simulink model "fft_wideband_real"  (R2012b)
settings: Solver=ode45  StartTime=0.0  StopTime=19999  RelTol=1e-3
undefined symbols (not defined in the file): fft_wideband_real_shift_schedule_user_data_out
libraries: xbsIndex_r4 x8703, xbsReplacements_r4 x36, xps_library x24, dspsigops x16, simulink_xsg_bridge x1
(part 9 of 51)

== system fft_wideband_real/fft_wideband_real/phase_mult/phase3_coeffs ==
  rst : Inport
  Counter : xbsIndex_r4/Counter  cnt_type=Free Running  cnt_to=Inf  operation=Up  start_count=0  cnt_by_val=1  arith_type=Unsigned  n_bits=6  bin_pt=0  load_pin=off  rst=on  en=off  explicit_period=on  period=1  dbl_ovrd=off  use_behavioral_HDL=off  implementation=Fabric  block_type=counter
  Slice : xbsIndex_r4/Slice  nbits=6  boolean_output=off  mode=Upper Bit Location + Width  bit1=0  base1=MSB of Input  bit0=0  base0=LSB of Input  dbl_ovrd=off  block_type=slice
  bram_din_const : xbsIndex_r4/Constant  const=0  gui_display_data_type=Fixed-point  arith_type=Signed (2's comp)  n_bits=18  bin_pt=17  preci_type=Single  exp_width=8  frac_width=24  explicit_period=off  period=1  equ=P=C  opselect=C  inp2=PCIN>>17  opr=+  inp1=P  carry=CIN  dbl_ovrd=off  block_type=constant
  bram_we_const : xbsIndex_r4/Constant  const=0  gui_display_data_type=Fixed-point  arith_type=Boolean  n_bits=16  bin_pt=14  preci_type=Single  exp_width=8  frac_width=24  explicit_period=off  period=1  equ=P=C  opselect=C  inp2=PCIN>>17  opr=+  inp1=P  carry=CIN  dbl_ovrd=off  block_type=constant
  cnt_sign_exta : xbsIndex_r4/Convert  gui_display_data_type=Fixed-point  arith_type=Unsigned  n_bits=10  bin_pt=0  float_type=Single  exp_bits=8  fraction_bits=24  quantization=Truncate  overflow=Wrap  en=off  latency=0  dbl_ovrd=off  pipeline=off  block_type=convert
  cnt_sign_extb : xbsIndex_r4/Convert  gui_display_data_type=Fixed-point  arith_type=Unsigned  n_bits=9  bin_pt=0  float_type=Single  exp_bits=8  fraction_bits=24  quantization=Truncate  overflow=Wrap  en=off  latency=0  dbl_ovrd=off  pipeline=off  block_type=convert
  coeff_mem : xbsIndex_r4/Dual Port RAM  depth=1024  initVector=[1 0.999923706054688 0.999702453613281 0.999320983886719 0.998794555664062 0.998115539550781 0.997291564941406 0.996315002441406 0.995185852050781 0.993904113769531 0.992477416992188 0.99090576171875 0.989173889160156 0.9873046875 0.985275268554688 0.983108520507812 0.980781555175781 0.978317260742188 0.975700378417969 0.972938537597656 0.97003173828125 0.96697998046875 0.963775634765625 0.960433959960938 0.956939697265625 0.95330810546875 0.949531555175781 0.945610046386719 0.941543579101562 0.937339782714844 0.932991027832031 0.928504943847656 0.923881530761719 0.919113159179688 0.914207458496094 0.909164428710938 0.90399169921875 0.898674011230469 0.893226623535156 0.887641906738281 0.881919860839844 0.876068115234375 0.870086669921875 0.863975524902344 0.85772705078125 0.851356506347656 0.844856262207031 0.838226318359375 0.831466674804688 0.824592590332031 0.817581176757812 0.810455322265625 0.803207397460938 0.79583740234375 0.788345336914062 0.780738830566406 0.77301025390625 0.765167236328125 0.757209777832031 0.749137878417969 0.740951538085938 0.732650756835938 0.724250793457031 0.715728759765625 0 0 0 0 0 0 0 0 0 0 0 0 0 0 0 0 0 0 0 0 0 0 0 0 0 0 0 0 0 0 0 0 0 0 0 0 0 0 0 0 0 0 0 0 0 0 0 0 0 0 0 0 0 0 0 0 0 0 0 0 0 0 0 0 0 0 0 0 0 0 0 0 0 0 0 0 0 0 0 0 0 0 0 0 0 0 0 0 0 0 0 0 0 0 0 0 0 0 0 0 0 0 0 0 0 0 0 0 0 0 0 0 0 0 0 0 0 0 0 0 0 0 0 0 0 0 0 0 0 0 0 0 0 0 0 0 0 0 0 0 0 0 0 0 0 0 0 0 0 0 0 0 0 0 0 0 0 0 0 0 0 0 0 0 0 0 0 0 0 0 0 0 0 0 0 0 0 0 0 0 0 0 0 0 0 0 0 0 0 0 0 0 0 0 0 0 0 0 0 0 0 0 0 0 0 0 0 0 0 0 0 0 0 0 0 0 0 0 0 0 0 0 0 0 0 0 0 0 0 0 0 0 0 0 0 0 0 0 0 0 0 0 0 0 0 0 0 0 0 0 0 0 0 0 0 0 0 0 0 0 0 0 0 0 0 0 0 0 0 0 0 0 0 0 0 0 0 0 0 0 0 0 0 0 0 0 0 0 0 0 0 0 0 0 0 0 0 0 0 0 0 0 0 0 0 0 0 0 0 0 0 0 0 0 0 0 0 0 0 0 0 0 0 0 0 0 0 0 0 0 0 0 0 0 0 0 0 0 0 0 0 0 0 0 0 0 0 0 0 0 0 0 0 0 0 0 0 0 0 0 0 0 0 0 0 0 0 0 0 0 0 0 0 0 0 0 0 0 0 0 0 0 0 0 0 0 0 0 0 0 0 0 0 0 0 0 0 0 0 0 0 0 0 0 0 0 0 0 0 0 0 0 0 0 0 0 0 0 0 0 0 0 0 0 0 0 0 0 0 0 0 0 0 0 0 0 0 0 0 0 0 0 0 0 0 0 0 0 0 -0.01226806640625 -0.0245437622070312 -0.03680419921875 -0.0490646362304688 -0.0613174438476562 -0.0735626220703125 -0.0858001708984375 -0.0980148315429688 -0.110221862792969 -0.122413635253906 -0.13458251953125 -0.146728515625 -0.158859252929688 -0.17095947265625 -0.183036804199219 -0.195091247558594 -0.207115173339844 -0.219100952148438 -0.231056213378906 -0.24298095703125 -0.254867553710938 -0.266716003417969 -0.278518676757812 -0.290283203125 -0.302009582519531 -0.313682556152344 -0.325309753417969 -0.336891174316406 -0.348419189453125 -0.359893798828125 -0.371315002441406 -0.382682800292969 -0.393989562988281 -0.405242919921875 -0.416427612304688 -0.427558898925781 -0.438613891601562 -0.449607849121094 -0.460540771484375 -0.471397399902344 -0.482185363769531 -0.492897033691406 -0.5035400390625 -0.51409912109375 -0.524589538574219 -0.534996032714844 -0.545326232910156 -0.555572509765625 -0.56573486328125 -0.5758056640625 -0.585800170898438 -0.595695495605469 -0.605514526367188 -0.615234375 -0.624862670898438 -0.634391784667969 -0.643829345703125 -0.653175354003906 -0.66241455078125 -0.671562194824219 -0.68060302734375 -0.689537048339844 -0.698379516601562 0 0 0 0 0 0 0 0 0 0 0 0 0 0 0 0 0 0 0 0 0 0 0 0 0 0 0 0 0 0 0 0 0 0 0 0 0 0 0 0 0 0 0 0 0 0 0 0 0 0 0 0 0 0 0 0 0 0 0 0 0 0 0 0 0 0 0 0 0 0 0 0 0 0 0 0 0 0 0 0 0 0 0 0 0 0 0 0 0 0 0 0 0 0 0 0 0 0 0 0 0 0 0 0 0 0 0 0 0 0 0 0 0 0 0 0 0 0 0 0 0 0 0 0 0 0 0 0 0 0 0 0 0 0 0 0 0 0 0 0 0 0 0 0 0 0 0 0 0 0 0 0 0 0 0 0 0 0 0 0 0 0 0 0 0 0 0 0 0 0 0 0 0 0 0 0 0 0 0 0 0 0 0 0 0 0 0 0 0 0 0 0 0 0 0 0 0 0 0 0 0 0 0 0 0 0 0 0 0 0 0 0 0 0 0 0 0 0 0 0 0 0 0 0 0 0 0 0 0 0 0 0 0 0 0 0 0 0 0 0 0 0 0 0 0 0 0 0 0 0 0 0 0 0 0 0 0 0 0 0 0 0 0 0 0 0 0 0 0 0 0 0 0 0 0 0 0 0 0 0 0 0 0 0 0 0 0 0 0 0 0 0 0 0 0 0 0 0 0 0 0 0 0 0 0 0 0 0 0 0 0 0 0 0 0 0 0 0 0 0 0 0 0 0 0 0 0 0 0 0 0 0 0 0 0 0 0 0 0 0 0 0 0 0 0 0 0 0 0 0 0 0 0 0 0 0 0 0 0 0 0 0 0 0 0 0 0 0 0 0 0 0 0 0 0 0 0 0 0 0 0 0 0 0 0 0 0 0 0 0 0 0 0 0 0 0 0 0 0 0 0 0 0 0 0 0 0 0 0 0 0 0 0 0 0 0 0 0 0 0 0 0 0 0 0 0 0 0 0 0 0 0 0 0 0 0 0 0 0 0 0 0 0 0 0 0 0 0]  distributed_mem=Block RAM  init_a=0  init_b=0  rst_a=off  rst_b=off  en_a=off  en_b=off  latency=2  write_mode_A=Read After Write  write_mode_B=Read After Write  dbl_ovrd=off  optimize=Area  use_rpm=on  block_type=dpram
  counter_b_concat : xbsIndex_r4/Concat  num_inputs=2  dbl_ovrd=off  block_type=concat
  counter_b_pad : xbsIndex_r4/Constant  const=1  gui_display_data_type=Fixed-point  arith_type=Unsigned  n_bits=1  bin_pt=0  preci_type=Single  exp_width=8  frac_width=24  explicit_period=off  period=1  equ=P=C  opselect=C  inp2=PCIN>>17  opr=+  inp1=P  carry=CIN  dbl_ovrd=off  block_type=constant
  ri_to_c : Subsystem
  w : Outport
  wires:
  Slice/1 -> cnt_sign_extb/1, cnt_sign_exta/1
  bram_din_const/1 -> coeff_mem/5, coeff_mem/2
  bram_we_const/1 -> coeff_mem/6, coeff_mem/3
  ri_to_c/1(c) -> w/1
  coeff_mem/2 -> ri_to_c/2(im)
  coeff_mem/1 -> ri_to_c/1(re)
  counter_b_concat/1 -> coeff_mem/4
  cnt_sign_exta/1 -> coeff_mem/1
  cnt_sign_extb/1 -> counter_b_concat/2
  counter_b_pad/1 -> counter_b_concat/1
  Counter/1 -> Slice/1
  rst/1 -> Counter/1

== system fft_wideband_real/fft_wideband_real/phase_mult/phase4_coeffs ==
  rst : Inport
  Counter : xbsIndex_r4/Counter  cnt_type=Free Running  cnt_to=Inf  operation=Up  start_count=0  cnt_by_val=1  arith_type=Unsigned  n_bits=6  bin_pt=0  load_pin=off  rst=on  en=off  explicit_period=on  period=1  dbl_ovrd=off  use_behavioral_HDL=off  implementation=Fabric  block_type=counter
  Slice : xbsIndex_r4/Slice  nbits=6  boolean_output=off  mode=Upper Bit Location + Width  bit1=0  base1=MSB of Input  bit0=0  base0=LSB of Input  dbl_ovrd=off  block_type=slice
  bram_din_const : xbsIndex_r4/Constant  const=0  gui_display_data_type=Fixed-point  arith_type=Signed (2's comp)  n_bits=18  bin_pt=17  preci_type=Single  exp_width=8  frac_width=24  explicit_period=off  period=1  equ=P=C  opselect=C  inp2=PCIN>>17  opr=+  inp1=P  carry=CIN  dbl_ovrd=off  block_type=constant
  bram_we_const : xbsIndex_r4/Constant  const=0  gui_display_data_type=Fixed-point  arith_type=Boolean  n_bits=16  bin_pt=14  preci_type=Single  exp_width=8  frac_width=24  explicit_period=off  period=1  equ=P=C  opselect=C  inp2=PCIN>>17  opr=+  inp1=P  carry=CIN  dbl_ovrd=off  block_type=constant
  cnt_sign_exta : xbsIndex_r4/Convert  gui_display_data_type=Fixed-point  arith_type=Unsigned  n_bits=10  bin_pt=0  float_type=Single  exp_bits=8  fraction_bits=24  quantization=Truncate  overflow=Wrap  en=off  latency=0  dbl_ovrd=off  pipeline=off  block_type=convert
  cnt_sign_extb : xbsIndex_r4/Convert  gui_display_data_type=Fixed-point  arith_type=Unsigned  n_bits=9  bin_pt=0  float_type=Single  exp_bits=8  fraction_bits=24  quantization=Truncate  overflow=Wrap  en=off  latency=0  dbl_ovrd=off  pipeline=off  block_type=convert
  coeff_mem : xbsIndex_r4/Dual Port RAM  depth=1024  initVector=[1 0.999832153320312 0.999320983886719 0.99847412109375 0.997291564941406 0.995765686035156 0.993904113769531 0.991706848144531 0.989173889160156 0.986305236816406 0.983108520507812 0.979568481445312 0.975700378417969 0.971504211425781 0.96697998046875 0.962120056152344 0.956939697265625 0.951431274414062 0.945610046386719 0.939460754394531 0.932991027832031 0.92620849609375 0.919113159179688 0.911705017089844 0.90399169921875 0.895965576171875 0.887641906738281 0.879013061523438 0.870086669921875 0.860870361328125 0.851356506347656 0.841552734375 0.831466674804688 0.82110595703125 0.810455322265625 0.799537658691406 0.788345336914062 0.776885986328125 0.765167236328125 0.753189086914062 0.740951538085938 0.728462219238281 0.715728759765625 0.702751159667969 0.689537048339844 0.676094055175781 0.66241455078125 0.648513793945312 0.634391784667969 0.62005615234375 0.605514526367188 0.59075927734375 0.5758056640625 0.560661315917969 0.545326232910156 0.529800415039062 0.51409912109375 0.49822998046875 0.482185363769531 0.465972900390625 0.449607849121094 0.433090209960938 0.416427612304688 0.399627685546875 0 0 0 0 0 0 0 0 0 0 0 0 0 0 0 0 0 0 0 0 0 0 0 0 0 0 0 0 0 0 0 0 0 0 0 0 0 0 0 0 0 0 0 0 0 0 0 0 0 0 0 0 0 0 0 0 0 0 0 0 0 0 0 0 0 0 0 0 0 0 0 0 0 0 0 0 0 0 0 0 0 0 0 0 0 0 0 0 0 0 0 0 0 0 0 0 0 0 0 0 0 0 0 0 0 0 0 0 0 0 0 0 0 0 0 0 0 0 0 0 0 0 0 0 0 0 0 0 0 0 0 0 0 0 0 0 0 0 0 0 0 0 0 0 0 0 0 0 0 0 0 0 0 0 0 0 0 0 0 0 0 0 0 0 0 0 0 0 0 0 0 0 0 0 0 0 0 0 0 0 0 0 0 0 0 0 0 0 0 0 0 0 0 0 0 0 0 0 0 0 0 0 0 0 0 0 0 0 0 0 0 0 0 0 0 0 0 0 0 0 0 0 0 0 0 0 0 0 0 0 0 0 0 0 0 0 0 0 0 0 0 0 0 0 0 0 0 0 0 0 0 0 0 0 0 0 0 0 0 0 0 0 0 0 0 0 0 0 0 0 0 0 0 0 0 0 0 0 0 0 0 0 0 0 0 0 0 0 0 0 0 0 0 0 0 0 0 0 0 0 0 0 0 0 0 0 0 0 0 0 0 0 0 0 0 0 0 0 0 0 0 0 0 0 0 0 0 0 0 0 0 0 0 0 0 0 0 0 0 0 0 0 0 0 0 0 0 0 0 0 0 0 0 0 0 0 0 0 0 0 0 0 0 0 0 0 0 0 0 0 0 0 0 0 0 0 0 0 0 0 0 0 0 0 0 0 0 0 0 0 0 0 0 0 0 0 0 0 0 0 0 0 0 0 0 0 0 0 0 0 0 0 0 0 0 0 0 0 0 0 0 0 0 0 0 0 0 0 0 0 0 0 0 0 0 0 0 0 0 0 0 0 0 0 0 0 0 0 0 -0.0184097290039062 -0.03680419921875 -0.0551986694335938 -0.0735626220703125 -0.0919113159179688 -0.110221862792969 -0.128501892089844 -0.146728515625 -0.164909362792969 -0.183036804199219 -0.201103210449219 -0.219100952148438 -0.237022399902344 -0.254867553710938 -0.272621154785156 -0.290283203125 -0.307846069335938 -0.325309753417969 -0.342658996582031 -0.359893798828125 -0.377006530761719 -0.393989562988281 -0.410842895507812 -0.427558898925781 -0.444122314453125 -0.460540771484375 -0.476799011230469 -0.492897033691406 -0.508827209472656 -0.524589538574219 -0.540168762207031 -0.555572509765625 -0.570777893066406 -0.585800170898438 -0.600616455078125 -0.615234375 -0.629638671875 -0.643829345703125 -0.657806396484375 -0.671562194824219 -0.685081481933594 -0.698379516601562 -0.711433410644531 -0.724250793457031 -0.73681640625 -0.749137878417969 -0.761199951171875 -0.77301025390625 -0.784553527832031 -0.79583740234375 -0.806846618652344 -0.817581176757812 -0.828048706054688 -0.838226318359375 -0.848121643066406 -0.85772705078125 -0.867042541503906 -0.876068115234375 -0.884796142578125 -0.893226623535156 -0.901351928710938 -0.909164428710938 -0.916679382324219 0 0 0 0 0 0 0 0 0 0 0 0 0 0 0 0 0 0 0 0 0 0 0 0 0 0 0 0 0 0 0 0 0 0 0 0 0 0 0 0 0 0 0 0 0 0 0 0 0 0 0 0 0 0 0 0 0 0 0 0 0 0 0 0 0 0 0 0 0 0 0 0 0 0 0 0 0 0 0 0 0 0 0 0 0 0 0 0 0 0 0 0 0 0 0 0 0 0 0 0 0 0 0 0 0 0 0 0 0 0 0 0 0 0 0 0 0 0 0 0 0 0 0 0 0 0 0 0 0 0 0 0 0 0 0 0 0 0 0 0 0 0 0 0 0 0 0 0 0 0 0 0 0 0 0 0 0 0 0 0 0 0 0 0 0 0 0 0 0 0 0 0 0 0 0 0 0 0 0 0 0 0 0 0 0 0 0 0 0 0 0 0 0 0 0 0 0 0 0 0 0 0 0 0 0 0 0 0 0 0 0 0 0 0 0 0 0 0 0 0 0 0 0 0 0 0 0 0 0 0 0 0 0 0 0 0 0 0 0 0 0 0 0 0 0 0 0 0 0 0 0 0 0 0 0 0 0 0 0 0 0 0 0 0 0 0 0 0 0 0 0 0 0 0 0 0 0 0 0 0 0 0 0 0 0 0 0 0 0 0 0 0 0 0 0 0 0 0 0 0 0 0 0 0 0 0 0 0 0 0 0 0 0 0 0 0 0 0 0 0 0 0 0 0 0 0 0 0 0 0 0 0 0 0 0 0 0 0 0 0 0 0 0 0 0 0 0 0 0 0 0 0 0 0 0 0 0 0 0 0 0 0 0 0 0 0 0 0 0 0 0 0 0 0 0 0 0 0 0 0 0 0 0 0 0 0 0 0 0 0 0 0 0 0 0 0 0 0 0 0 0 0 0 0 0 0 0 0 0 0 0 0 0 0 0 0 0 0 0 0 0 0 0 0 0 0 0 0 0 0 0 0 0 0 0 0 0 0 0 0 0 0 0 0 0 0 0 0]  distributed_mem=Block RAM  init_a=0  init_b=0  rst_a=off  rst_b=off  en_a=off  en_b=off  latency=2  write_mode_A=Read After Write  write_mode_B=Read After Write  dbl_ovrd=off  optimize=Area  use_rpm=on  block_type=dpram
  counter_b_concat : xbsIndex_r4/Concat  num_inputs=2  dbl_ovrd=off  block_type=concat
  counter_b_pad : xbsIndex_r4/Constant  const=1  gui_display_data_type=Fixed-point  arith_type=Unsigned  n_bits=1  bin_pt=0  preci_type=Single  exp_width=8  frac_width=24  explicit_period=off  period=1  equ=P=C  opselect=C  inp2=PCIN>>17  opr=+  inp1=P  carry=CIN  dbl_ovrd=off  block_type=constant
  ri_to_c : Subsystem
  w : Outport
  wires:
  Slice/1 -> cnt_sign_extb/1, cnt_sign_exta/1
  bram_din_const/1 -> coeff_mem/5, coeff_mem/2
  bram_we_const/1 -> coeff_mem/6, coeff_mem/3
  ri_to_c/1(c) -> w/1
  coeff_mem/2 -> ri_to_c/2(im)
  coeff_mem/1 -> ri_to_c/1(re)
  counter_b_concat/1 -> coeff_mem/4
  cnt_sign_exta/1 -> coeff_mem/1
  cnt_sign_extb/1 -> counter_b_concat/2
  counter_b_pad/1 -> counter_b_concat/1
  Counter/1 -> Slice/1
  rst/1 -> Counter/1

== system fft_wideband_real/fft_wideband_real/phase_mult/phase5_coeffs ==
  rst : Inport
  Counter : xbsIndex_r4/Counter  cnt_type=Free Running  cnt_to=Inf  operation=Up  start_count=0  cnt_by_val=1  arith_type=Unsigned  n_bits=6  bin_pt=0  load_pin=off  rst=on  en=off  explicit_period=on  period=1  dbl_ovrd=off  use_behavioral_HDL=off  implementation=Fabric  block_type=counter
  Slice : xbsIndex_r4/Slice  nbits=6  boolean_output=off  mode=Upper Bit Location + Width  bit1=0  base1=MSB of Input  bit0=0  base0=LSB of Input  dbl_ovrd=off  block_type=slice
  bram_din_const : xbsIndex_r4/Constant  const=0  gui_display_data_type=Fixed-point  arith_type=Signed (2's comp)  n_bits=18  bin_pt=17  preci_type=Single  exp_width=8  frac_width=24  explicit_period=off  period=1  equ=P=C  opselect=C  inp2=PCIN>>17  opr=+  inp1=P  carry=CIN  dbl_ovrd=off  block_type=constant
  bram_we_const : xbsIndex_r4/Constant  const=0  gui_display_data_type=Fixed-point  arith_type=Boolean  n_bits=16  bin_pt=14  preci_type=Single  exp_width=8  frac_width=24  explicit_period=off  period=1  equ=P=C  opselect=C  inp2=PCIN>>17  opr=+  inp1=P  carry=CIN  dbl_ovrd=off  block_type=constant
  cnt_sign_exta : xbsIndex_r4/Convert  gui_display_data_type=Fixed-point  arith_type=Unsigned  n_bits=10  bin_pt=0  float_type=Single  exp_bits=8  fraction_bits=24  quantization=Truncate  overflow=Wrap  en=off  latency=0  dbl_ovrd=off  pipeline=off  block_type=convert
  cnt_sign_extb : xbsIndex_r4/Convert  gui_display_data_type=Fixed-point  arith_type=Unsigned  n_bits=9  bin_pt=0  float_type=Single  exp_bits=8  fraction_bits=24  quantization=Truncate  overflow=Wrap  en=off  latency=0  dbl_ovrd=off  pipeline=off  block_type=convert
  coeff_mem : xbsIndex_r4/Dual Port RAM  depth=1024  initVector=[1 0.999702453613281 0.998794555664062 0.997291564941406 0.995185852050781 0.992477416992188 0.989173889160156 0.985275268554688 0.980781555175781 0.975700378417969 0.97003173828125 0.963775634765625 0.956939697265625 0.949531555175781 0.941543579101562 0.932991027832031 0.923881530761719 0.914207458496094 0.90399169921875 0.893226623535156 0.881919860839844 0.870086669921875 0.85772705078125 0.844856262207031 0.831466674804688 0.817581176757812 0.803207397460938 0.788345336914062 0.77301025390625 0.757209777832031 0.740951538085938 0.724250793457031 0.707107543945312 0.689537048339844 0.671562194824219 0.653175354003906 0.634391784667969 0.615234375 0.595695495605469 0.5758056640625 0.555572509765625 0.534996032714844 0.51409912109375 0.492897033691406 0.471397399902344 0.449607849121094 0.427558898925781 0.405242919921875 0.382682800292969 0.359893798828125 0.336891174316406 0.313682556152344 0.290283203125 0.266716003417969 0.24298095703125 0.219100952148438 0.195091247558594 0.17095947265625 0.146728515625 0.122413635253906 0.0980148315429688 0.0735626220703125 0.0490646362304688 0.0245437622070312 0 0 0 0 0 0 0 0 0 0 0 0 0 0 0 0 0 0 0 0 0 0 0 0 0 0 0 0 0 0 0 0 0 0 0 0 0 0 0 0 0 0 0 0 0 0 0 0 0 0 0 0 0 0 0 0 0 0 0 0 0 0 0 0 0 0 0 0 0 0 0 0 0 0 0 0 0 0 0 0 0 0 0 0 0 0 0 0 0 0 0 0 0 0 0 0 0 0 0 0 0 0 0 0 0 0 0 0 0 0 0 0 0 0 0 0 0 0 0 0 0 0 0 0 0 0 0 0 0 0 0 0 0 0 0 0 0 0 0 0 0 0 0 0 0 0 0 0 0 0 0 0 0 0 0 0 0 0 0 0 0 0 0 0 0 0 0 0 0 0 0 0 0 0 0 0 0 0 0 0 0 0 0 0 0 0 0 0 0 0 0 0 0 0 0 0 0 0 0 0 0 0 0 0 0 0 0 0 0 0 0 0 0 0 0 0 0 0 0 0 0 0 0 0 0 0 0 0 0 0 0 0 0 0 0 0 0 0 0 0 0 0 0 0 0 0 0 0 0 0 0 0 0 0 0 0 0 0 0 0 0 0 0 0 0 0 0 0 0 0 0 0 0 0 0 0 0 0 0 0 0 0 0 0 0 0 0 0 0 0 0 0 0 0 0 0 0 0 0 0 0 0 0 0 0 0 0 0 0 0 0 0 0 0 0 0 0 0 0 0 0 0 0 0 0 0 0 0 0 0 0 0 0 0 0 0 0 0 0 0 0 0 0 0 0 0 0 0 0 0 0 0 0 0 0 0 0 0 0 0 0 0 0 0 0 0 0 0 0 0 0 0 0 0 0 0 0 0 0 0 0 0 0 0 0 0 0 0 0 0 0 0 0 0 0 0 0 0 0 0 0 0 0 0 0 0 0 0 0 0 0 0 0 0 0 0 0 0 0 0 0 0 0 0 0 0 0 0 0 0 0 0 0 0 0 0 0 0 0 0 0 0 0 0 0 0 0 0 0 -0.0245437622070312 -0.0490646362304688 -0.0735626220703125 -0.0980148315429688 -0.122413635253906 -0.146728515625 -0.17095947265625 -0.195091247558594 -0.219100952148438 -0.24298095703125 -0.266716003417969 -0.290283203125 -0.313682556152344 -0.336891174316406 -0.359893798828125 -0.382682800292969 -0.405242919921875 -0.427558898925781 -0.449607849121094 -0.471397399902344 -0.492897033691406 -0.51409912109375 -0.534996032714844 -0.555572509765625 -0.5758056640625 -0.595695495605469 -0.615234375 -0.634391784667969 -0.653175354003906 -0.671562194824219 -0.689537048339844 -0.707107543945312 -0.724250793457031 -0.740951538085938 -0.757209777832031 -0.77301025390625 -0.788345336914062 -0.803207397460938 -0.817581176757812 -0.831466674804688 -0.844856262207031 -0.85772705078125 -0.870086669921875 -0.881919860839844 -0.893226623535156 -0.90399169921875 -0.914207458496094 -0.923881530761719 -0.932991027832031 -0.941543579101562 -0.949531555175781 -0.956939697265625 -0.963775634765625 -0.97003173828125 -0.975700378417969 -0.980781555175781 -0.985275268554688 -0.989173889160156 -0.992477416992188 -0.995185852050781 -0.997291564941406 -0.998794555664062 -0.999702453613281 0 0 0 0 0 0 0 0 0 0 0 0 0 0 0 0 0 0 0 0 0 0 0 0 0 0 0 0 0 0 0 0 0 0 0 0 0 0 0 0 0 0 0 0 0 0 0 0 0 0 0 0 0 0 0 0 0 0 0 0 0 0 0 0 0 0 0 0 0 0 0 0 0 0 0 0 0 0 0 0 0 0 0 0 0 0 0 0 0 0 0 0 0 0 0 0 0 0 0 0 0 0 0 0 0 0 0 0 0 0 0 0 0 0 0 0 0 0 0 0 0 0 0 0 0 0 0 0 0 0 0 0 0 0 0 0 0 0 0 0 0 0 0 0 0 0 0 0 0 0 0 0 0 0 0 0 0 0 0 0 0 0 0 0 0 0 0 0 0 0 0 0 0 0 0 0 0 0 0 0 0 0 0 0 0 0 0 0 0 0 0 0 0 0 0 0 0 0 0 0 0 0 0 0 0 0 0 0 0 0 0 0 0 0 0 0 0 0 0 0 0 0 0 0 0 0 0 0 0 0 0 0 0 0 0 0 0 0 0 0 0 0 0 0 0 0 0 0 0 0 0 0 0 0 0 0 0 0 0 0 0 0 0 0 0 0 0 0 0 0 0 0 0 0 0 0 0 0 0 0 0 0 0 0 0 0 0 0 0 0 0 0 0 0 0 0 0 0 0 0 0 0 0 0 0 0 0 0 0 0 0 0 0 0 0 0 0 0 0 0 0 0 0 0 0 0 0 0 0 0 0 0 0 0 0 0 0 0 0 0 0 0 0 0 0 0 0 0 0 0 0 0 0 0 0 0 0 0 0 0 0 0 0 0 0 0 0 0 0 0 0 0 0 0 0 0 0 0 0 0 0 0 0 0 0 0 0 0 0 0 0 0 0 0 0 0 0 0 0 0 0 0 0 0 0 0 0 0 0 0 0 0 0 0 0 0 0 0 0 0 0 0 0 0 0 0 0 0 0 0 0 0 0 0 0 0 0 0 0 0 0 0 0 0 0 0 0 0]  distributed_mem=Block RAM  init_a=0  init_b=0  rst_a=off  rst_b=off  en_a=off  en_b=off  latency=2  write_mode_A=Read After Write  write_mode_B=Read After Write  dbl_ovrd=off  optimize=Area  use_rpm=on  block_type=dpram
  counter_b_concat : xbsIndex_r4/Concat  num_inputs=2  dbl_ovrd=off  block_type=concat
  counter_b_pad : xbsIndex_r4/Constant  const=1  gui_display_data_type=Fixed-point  arith_type=Unsigned  n_bits=1  bin_pt=0  preci_type=Single  exp_width=8  frac_width=24  explicit_period=off  period=1  equ=P=C  opselect=C  inp2=PCIN>>17  opr=+  inp1=P  carry=CIN  dbl_ovrd=off  block_type=constant
  ri_to_c : Subsystem
  w : Outport
  wires:
  Slice/1 -> cnt_sign_extb/1, cnt_sign_exta/1
  bram_din_const/1 -> coeff_mem/5, coeff_mem/2
  bram_we_const/1 -> coeff_mem/6, coeff_mem/3
  ri_to_c/1(c) -> w/1
  coeff_mem/2 -> ri_to_c/2(im)
  coeff_mem/1 -> ri_to_c/1(re)
  counter_b_concat/1 -> coeff_mem/4
  cnt_sign_exta/1 -> coeff_mem/1
  cnt_sign_extb/1 -> counter_b_concat/2
  counter_b_pad/1 -> counter_b_concat/1
  Counter/1 -> Slice/1
  rst/1 -> Counter/1

== system fft_wideband_real/fft_wideband_real/phase_mult/phase6_coeffs ==
  rst : Inport
  Counter : xbsIndex_r4/Counter  cnt_type=Free Running  cnt_to=Inf  operation=Up  start_count=0  cnt_by_val=1  arith_type=Unsigned  n_bits=6  bin_pt=0  load_pin=off  rst=on  en=off  explicit_period=on  period=1  dbl_ovrd=off  use_behavioral_HDL=off  implementation=Fabric  block_type=counter
  Slice : xbsIndex_r4/Slice  nbits=6  boolean_output=off  mode=Upper Bit Location + Width  bit1=0  base1=MSB of Input  bit0=0  base0=LSB of Input  dbl_ovrd=off  block_type=slice
  bram_din_const : xbsIndex_r4/Constant  const=0  gui_display_data_type=Fixed-point  arith_type=Signed (2's comp)  n_bits=18  bin_pt=17  preci_type=Single  exp_width=8  frac_width=24  explicit_period=off  period=1  equ=P=C  opselect=C  inp2=PCIN>>17  opr=+  inp1=P  carry=CIN  dbl_ovrd=off  block_type=constant
  bram_we_const : xbsIndex_r4/Constant  const=0  gui_display_data_type=Fixed-point  arith_type=Boolean  n_bits=16  bin_pt=14  preci_type=Single  exp_width=8  frac_width=24  explicit_period=off  period=1  equ=P=C  opselect=C  inp2=PCIN>>17  opr=+  inp1=P  carry=CIN  dbl_ovrd=off  block_type=constant
  cnt_sign_exta : xbsIndex_r4/Convert  gui_display_data_type=Fixed-point  arith_type=Unsigned  n_bits=10  bin_pt=0  float_type=Single  exp_bits=8  fraction_bits=24  quantization=Truncate  overflow=Wrap  en=off  latency=0  dbl_ovrd=off  pipeline=off  block_type=convert
  cnt_sign_extb : xbsIndex_r4/Convert  gui_display_data_type=Fixed-point  arith_type=Unsigned  n_bits=9  bin_pt=0  float_type=Single  exp_bits=8  fraction_bits=24  quantization=Truncate  overflow=Wrap  en=off  latency=0  dbl_ovrd=off  pipeline=off  block_type=convert
  coeff_mem : xbsIndex_r4/Dual Port RAM  depth=1024  initVector=[1 0.999526977539062 0.998115539550781 0.995765686035156 0.992477416992188 0.988258361816406 0.983108520507812 0.977027893066406 0.97003173828125 0.962120056152344 0.95330810546875 0.943595886230469 0.932991027832031 0.921516418457031 0.909164428710938 0.895965576171875 0.881919860839844 0.867042541503906 0.851356506347656 0.834861755371094 0.817581176757812 0.799537658691406 0.780738830566406 0.761199951171875 0.740951538085938 0.720001220703125 0.698379516601562 0.676094055175781 0.653175354003906 0.629638671875 0.605514526367188 0.580810546875 0.555572509765625 0.529800415039062 0.5035400390625 0.476799011230469 0.449607849121094 0.4219970703125 0.393989562988281 0.365615844726562 0.336891174316406 0.307846069335938 0.278518676757812 0.248924255371094 0.219100952148438 0.189071655273438 0.158859252929688 0.128501892089844 0.0980148315429688 0.06744384765625 0.03680419921875 0.006134033203125 -0.0245437622070312 -0.0551986694335938 -0.0858001708984375 -0.116317749023438 -0.146728515625 -0.177001953125 -0.207115173339844 -0.237022399902344 -0.266716003417969 -0.296150207519531 -0.325309753417969 -0.354164123535156 0 0 0 0 0 0 0 0 0 0 0 0 0 0 0 0 0 0 0 0 0 0 0 0 0 0 0 0 0 0 0 0 0 0 0 0 0 0 0 0 0 0 0 0 0 0 0 0 0 0 0 0 0 0 0 0 0 0 0 0 0 0 0 0 0 0 0 0 0 0 0 0 0 0 0 0 0 0 0 0 0 0 0 0 0 0 0 0 0 0 0 0 0 0 0 0 0 0 0 0 0 0 0 0 0 0 0 0 0 0 0 0 0 0 0 0 0 0 0 0 0 0 0 0 0 0 0 0 0 0 0 0 0 0 0 0 0 0 0 0 0 0 0 0 0 0 0 0 0 0 0 0 0 0 0 0 0 0 0 0 0 0 0 0 0 0 0 0 0 0 0 0 0 0 0 0 0 0 0 0 0 0 0 0 0 0 0 0 0 0 0 0 0 0 0 0 0 0 0 0 0 0 0 0 0 0 0 0 0 0 0 0 0 0 0 0 0 0 0 0 0 0 0 0 0 0 0 0 0 0 0 0 0 0 0 0 0 0 0 0 0 0 0 0 0 0 0 0 0 0 0 0 0 0 0 0 0 0 0 0 0 0 0 0 0 0 0 0 0 0 0 0 0 0 0 0 0 0 0 0 0 0 0 0 0 0 0 0 0 0 0 0 0 0 0 0 0 0 0 0 0 0 0 0 0 0 0 0 0 0 0 0 0 0 0 0 0 0 0 0 0 0 0 0 0 0 0 0 0 0 0 0 0 0 0 0 0 0 0 0 0 0 0 0 0 0 0 0 0 0 0 0 0 0 0 0 0 0 0 0 0 0 0 0 0 0 0 0 0 0 0 0 0 0 0 0 0 0 0 0 0 0 0 0 0 0 0 0 0 0 0 0 0 0 0 0 0 0 0 0 0 0 0 0 0 0 0 0 0 0 0 0 0 0 0 0 0 0 0 0 0 0 0 0 0 0 0 0 0 0 0 0 0 0 0 0 0 0 0 0 0 0 0 0 0 0 0 0 0 -0.0306777954101562 -0.0613174438476562 -0.0919113159179688 -0.122413635253906 -0.152793884277344 -0.183036804199219 -0.213111877441406 -0.24298095703125 -0.272621154785156 -0.302009582519531 -0.331108093261719 -0.359893798828125 -0.388343811035156 -0.416427612304688 -0.444122314453125 -0.471397399902344 -0.49822998046875 -0.524589538574219 -0.550460815429688 -0.5758056640625 -0.600616455078125 -0.624862670898438 -0.648513793945312 -0.671562194824219 -0.6939697265625 -0.715728759765625 -0.73681640625 -0.757209777832031 -0.776885986328125 -0.79583740234375 -0.814033508300781 -0.831466674804688 -0.848121643066406 -0.863975524902344 -0.879013061523438 -0.893226623535156 -0.906593322753906 -0.919113159179688 -0.930763244628906 -0.941543579101562 -0.951431274414062 -0.960433959960938 -0.968521118164062 -0.975700378417969 -0.981964111328125 -0.9873046875 -0.991706848144531 -0.995185852050781 -0.997726440429688 -0.999320983886719 -0.999984741210938 -0.999702453613281 -0.99847412109375 -0.996315002441406 -0.993209838867188 -0.989173889160156 -0.984207153320312 -0.978317260742188 -0.971504211425781 -0.963775634765625 -0.95513916015625 -0.945610046386719 -0.9351806640625 0 0 0 0 0 0 0 0 0 0 0 0 0 0 0 0 0 0 0 0 0 0 0 0 0 0 0 0 0 0 0 0 0 0 0 0 0 0 0 0 0 0 0 0 0 0 0 0 0 0 0 0 0 0 0 0 0 0 0 0 0 0 0 0 0 0 0 0 0 0 0 0 0 0 0 0 0 0 0 0 0 0 0 0 0 0 0 0 0 0 0 0 0 0 0 0 0 0 0 0 0 0 0 0 0 0 0 0 0 0 0 0 0 0 0 0 0 0 0 0 0 0 0 0 0 0 0 0 0 0 0 0 0 0 0 0 0 0 0 0 0 0 0 0 0 0 0 0 0 0 0 0 0 0 0 0 0 0 0 0 0 0 0 0 0 0 0 0 0 0 0 0 0 0 0 0 0 0 0 0 0 0 0 0 0 0 0 0 0 0 0 0 0 0 0 0 0 0 0 0 0 0 0 0 0 0 0 0 0 0 0 0 0 0 0 0 0 0 0 0 0 0 0 0 0 0 0 0 0 0 0 0 0 0 0 0 0 0 0 0 0 0 0 0 0 0 0 0 0 0 0 0 0 0 0 0 0 0 0 0 0 0 0 0 0 0 0 0 0 0 0 0 0 0 0 0 0 0 0 0 0 0 0 0 0 0 0 0 0 0 0 0 0 0 0 0 0 0 0 0 0 0 0 0 0 0 0 0 0 0 0 0 0 0 0 0 0 0 0 0 0 0 0 0 0 0 0 0 0 0 0 0 0 0 0 0 0 0 0 0 0 0 0 0 0 0 0 0 0 0 0 0 0 0 0 0 0 0 0 0 0 0 0 0 0 0 0 0 0 0 0 0 0 0 0 0 0 0 0 0 0 0 0 0 0 0 0 0 0 0 0 0 0 0 0 0 0 0 0 0 0 0 0 0 0 0 0 0 0 0 0 0 0 0 0 0 0 0 0 0 0 0 0 0 0 0 0 0 0 0 0 0 0 0 0 0 0 0 0 0 0 0 0 0 0 0 0 0]  distributed_mem=Block RAM  init_a=0  init_b=0  rst_a=off  rst_b=off  en_a=off  en_b=off  latency=2  write_mode_A=Read After Write  write_mode_B=Read After Write  dbl_ovrd=off  optimize=Area  use_rpm=on  block_type=dpram
  counter_b_concat : xbsIndex_r4/Concat  num_inputs=2  dbl_ovrd=off  block_type=concat
  counter_b_pad : xbsIndex_r4/Constant  const=1  gui_display_data_type=Fixed-point  arith_type=Unsigned  n_bits=1  bin_pt=0  preci_type=Single  exp_width=8  frac_width=24  explicit_period=off  period=1  equ=P=C  opselect=C  inp2=PCIN>>17  opr=+  inp1=P  carry=CIN  dbl_ovrd=off  block_type=constant
  ri_to_c : Subsystem
  w : Outport
  wires:
  Slice/1 -> cnt_sign_extb/1, cnt_sign_exta/1
  bram_din_const/1 -> coeff_mem/5, coeff_mem/2
  bram_we_const/1 -> coeff_mem/6, coeff_mem/3
  ri_to_c/1(c) -> w/1
  coeff_mem/2 -> ri_to_c/2(im)
  coeff_mem/1 -> ri_to_c/1(re)
  counter_b_concat/1 -> coeff_mem/4
  cnt_sign_exta/1 -> coeff_mem/1
  cnt_sign_extb/1 -> counter_b_concat/2
  counter_b_pad/1 -> counter_b_concat/1
  Counter/1 -> Slice/1
  rst/1 -> Counter/1

== system fft_wideband_real/fft_wideband_real/phase_mult/phase7_coeffs ==
  rst : Inport
  Counter : xbsIndex_r4/Counter  cnt_type=Free Running  cnt_to=Inf  operation=Up  start_count=0  cnt_by_val=1  arith_type=Unsigned  n_bits=6  bin_pt=0  load_pin=off  rst=on  en=off  explicit_period=on  period=1  dbl_ovrd=off  use_behavioral_HDL=off  implementation=Fabric  block_type=counter
  Slice : xbsIndex_r4/Slice  nbits=6  boolean_output=off  mode=Upper Bit Location + Width  bit1=0  base1=MSB of Input  bit0=0  base0=LSB of Input  dbl_ovrd=off  block_type=slice
  bram_din_const : xbsIndex_r4/Constant  const=0  gui_display_data_type=Fixed-point  arith_type=Signed (2's comp)  n_bits=18  bin_pt=17  preci_type=Single  exp_width=8  frac_width=24  explicit_period=off  period=1  equ=P=C  opselect=C  inp2=PCIN>>17  opr=+  inp1=P  carry=CIN  dbl_ovrd=off  block_type=constant
  bram_we_const : xbsIndex_r4/Constant  const=0  gui_display_data_type=Fixed-point  arith_type=Boolean  n_bits=16  bin_pt=14  preci_type=Single  exp_width=8  frac_width=24  explicit_period=off  period=1  equ=P=C  opselect=C  inp2=PCIN>>17  opr=+  inp1=P  carry=CIN  dbl_ovrd=off  block_type=constant
  cnt_sign_exta : xbsIndex_r4/Convert  gui_display_data_type=Fixed-point  arith_type=Unsigned  n_bits=10  bin_pt=0  float_type=Single  exp_bits=8  fraction_bits=24  quantization=Truncate  overflow=Wrap  en=off  latency=0  dbl_ovrd=off  pipeline=off  block_type=convert
  cnt_sign_extb : xbsIndex_r4/Convert  gui_display_data_type=Fixed-point  arith_type=Unsigned  n_bits=9  bin_pt=0  float_type=Single  exp_bits=8  fraction_bits=24  quantization=Truncate  overflow=Wrap  en=off  latency=0  dbl_ovrd=off  pipeline=off  block_type=convert
  coeff_mem : xbsIndex_r4/Dual Port RAM  depth=1024  initVector=[1 0.999320983886719 0.997291564941406 0.993904113769531 0.989173889160156 0.983108520507812 0.975700378417969 0.96697998046875 0.956939697265625 0.945610046386719 0.932991027832031 0.919113159179688 0.90399169921875 0.887641906738281 0.870086669921875 0.851356506347656 0.831466674804688 0.810455322265625 0.788345336914062 0.765167236328125 0.740951538085938 0.715728759765625 0.689537048339844 0.66241455078125 0.634391784667969 0.605514526367188 0.5758056640625 0.545326232910156 0.51409912109375 0.482185363769531 0.449607849121094 0.416427612304688 0.382682800292969 0.348419189453125 0.313682556152344 0.278518676757812 0.24298095703125 0.207115173339844 0.17095947265625 0.13458251953125 0.0980148315429688 0.0613174438476562 0.0245437622070312 -0.01226806640625 -0.0490646362304688 -0.0858001708984375 -0.122413635253906 -0.158859252929688 -0.195091247558594 -0.231056213378906 -0.266716003417969 -0.302009582519531 -0.336891174316406 -0.371315002441406 -0.405242919921875 -0.438613891601562 -0.471397399902344 -0.5035400390625 -0.534996032714844 -0.56573486328125 -0.595695495605469 -0.624862670898438 -0.653175354003906 -0.68060302734375 0 0 0 0 0 0 0 0 0 0 0 0 0 0 0 0 0 0 0 0 0 0 0 0 0 0 0 0 0 0 0 0 0 0 0 0 0 0 0 0 0 0 0 0 0 0 0 0 0 0 0 0 0 0 0 0 0 0 0 0 0 0 0 0 0 0 0 0 0 0 0 0 0 0 0 0 0 0 0 0 0 0 0 0 0 0 0 0 0 0 0 0 0 0 0 0 0 0 0 0 0 0 0 0 0 0 0 0 0 0 0 0 0 0 0 0 0 0 0 0 0 0 0 0 0 0 0 0 0 0 0 0 0 0 0 0 0 0 0 0 0 0 0 0 0 0 0 0 0 0 0 0 0 0 0 0 0 0 0 0 0 0 0 0 0 0 0 0 0 0 0 0 0 0 0 0 0 0 0 0 0 0 0 0 0 0 0 0 0 0 0 0 0 0 0 0 0 0 0 0 0 0 0 0 0 0 0 0 0 0 0 0 0 0 0 0 0 0 0 0 0 0 0 0 0 0 0 0 0 0 0 0 0 0 0 0 0 0 0 0 0 0 0 0 0 0 0 0 0 0 0 0 0 0 0 0 0 0 0 0 0 0 0 0 0 0 0 0 0 0 0 0 0 0 0 0 0 0 0 0 0 0 0 0 0 0 0 0 0 0 0 0 0 0 0 0 0 0 0 0 0 0 0 0 0 0 0 0 0 0 0 0 0 0 0 0 0 0 0 0 0 0 0 0 0 0 0 0 0 0 0 0 0 0 0 0 0 0 0 0 0 0 0 0 0 0 0 0 0 0 0 0 0 0 0 0 0 0 0 0 0 0 0 0 0 0 0 0 0 0 0 0 0 0 0 0 0 0 0 0 0 0 0 0 0 0 0 0 0 0 0 0 0 0 0 0 0 0 0 0 0 0 0 0 0 0 0 0 0 0 0 0 0 0 0 0 0 0 0 0 0 0 0 0 0 0 0 0 0 0 0 0 0 0 0 0 0 0 0 0 0 0 0 0 0 0 0 0 0 -0.03680419921875 -0.0735626220703125 -0.110221862792969 -0.146728515625 -0.183036804199219 -0.219100952148438 -0.254867553710938 -0.290283203125 -0.325309753417969 -0.359893798828125 -0.393989562988281 -0.427558898925781 -0.460540771484375 -0.492897033691406 -0.524589538574219 -0.555572509765625 -0.585800170898438 -0.615234375 -0.643829345703125 -0.671562194824219 -0.698379516601562 -0.724250793457031 -0.749137878417969 -0.77301025390625 -0.79583740234375 -0.817581176757812 -0.838226318359375 -0.85772705078125 -0.876068115234375 -0.893226623535156 -0.909164428710938 -0.923881530761719 -0.937339782714844 -0.949531555175781 -0.960433959960938 -0.97003173828125 -0.978317260742188 -0.985275268554688 -0.99090576171875 -0.995185852050781 -0.998115539550781 -0.999702453613281 -0.999923706054688 -0.998794555664062 -0.996315002441406 -0.992477416992188 -0.9873046875 -0.980781555175781 -0.972938537597656 -0.963775634765625 -0.95330810546875 -0.941543579101562 -0.928504943847656 -0.914207458496094 -0.898674011230469 -0.881919860839844 -0.863975524902344 -0.844856262207031 -0.824592590332031 -0.803207397460938 -0.780738830566406 -0.757209777832031 -0.732650756835938 0 0 0 0 0 0 0 0 0 0 0 0 0 0 0 0 0 0 0 0 0 0 0 0 0 0 0 0 0 0 0 0 0 0 0 0 0 0 0 0 0 0 0 0 0 0 0 0 0 0 0 0 0 0 0 0 0 0 0 0 0 0 0 0 0 0 0 0 0 0 0 0 0 0 0 0 0 0 0 0 0 0 0 0 0 0 0 0 0 0 0 0 0 0 0 0 0 0 0 0 0 0 0 0 0 0 0 0 0 0 0 0 0 0 0 0 0 0 0 0 0 0 0 0 0 0 0 0 0 0 0 0 0 0 0 0 0 0 0 0 0 0 0 0 0 0 0 0 0 0 0 0 0 0 0 0 0 0 0 0 0 0 0 0 0 0 0 0 0 0 0 0 0 0 0 0 0 0 0 0 0 0 0 0 0 0 0 0 0 0 0 0 0 0 0 0 0 0 0 0 0 0 0 0 0 0 0 0 0 0 0 0 0 0 0 0 0 0 0 0 0 0 0 0 0 0 0 0 0 0 0 0 0 0 0 0 0 0 0 0 0 0 0 0 0 0 0 0 0 0 0 0 0 0 0 0 0 0 0 0 0 0 0 0 0 0 0 0 0 0 0 0 0 0 0 0 0 0 0 0 0 0 0 0 0 0 0 0 0 0 0 0 0 0 0 0 0 0 0 0 0 0 0 0 0 0 0 0 0 0 0 0 0 0 0 0 0 0 0 0 0 0 0 0 0 0 0 0 0 0 0 0 0 0 0 0 0 0 0 0 0 0 0 0 0 0 0 0 0 0 0 0 0 0 0 0 0 0 0 0 0 0 0 0 0 0 0 0 0 0 0 0 0 0 0 0 0 0 0 0 0 0 0 0 0 0 0 0 0 0 0 0 0 0 0 0 0 0 0 0 0 0 0 0 0 0 0 0 0 0 0 0 0 0 0 0 0 0 0 0 0 0 0 0 0 0 0 0 0 0 0 0 0 0 0 0 0 0 0 0 0 0 0 0 0 0 0 0]  distributed_mem=Block RAM  init_a=0  init_b=0  rst_a=off  rst_b=off  en_a=off  en_b=off  latency=2  write_mode_A=Read After Write  write_mode_B=Read After Write  dbl_ovrd=off  optimize=Area  use_rpm=on  block_type=dpram
  counter_b_concat : xbsIndex_r4/Concat  num_inputs=2  dbl_ovrd=off  block_type=concat
  counter_b_pad : xbsIndex_r4/Constant  const=1  gui_display_data_type=Fixed-point  arith_type=Unsigned  n_bits=1  bin_pt=0  preci_type=Single  exp_width=8  frac_width=24  explicit_period=off  period=1  equ=P=C  opselect=C  inp2=PCIN>>17  opr=+  inp1=P  carry=CIN  dbl_ovrd=off  block_type=constant
  ri_to_c : Subsystem
  w : Outport
  wires:
  Slice/1 -> cnt_sign_extb/1, cnt_sign_exta/1
  bram_din_const/1 -> coeff_mem/5, coeff_mem/2
  bram_we_const/1 -> coeff_mem/6, coeff_mem/3
  ri_to_c/1(c) -> w/1
  coeff_mem/2 -> ri_to_c/2(im)
  coeff_mem/1 -> ri_to_c/1(re)
  counter_b_concat/1 -> coeff_mem/4
  cnt_sign_exta/1 -> coeff_mem/1
  cnt_sign_extb/1 -> counter_b_concat/2
  counter_b_pad/1 -> counter_b_concat/1
  Counter/1 -> Slice/1
  rst/1 -> Counter/1

== system fft_wideband_real/fft_wideband_real/phase_mult/phase8_coeffs ==
  rst : Inport
  Counter : xbsIndex_r4/Counter  cnt_type=Free Running  cnt_to=Inf  operation=Up  start_count=0  cnt_by_val=1  arith_type=Unsigned  n_bits=6  bin_pt=0  load_pin=off  rst=on  en=off  explicit_period=on  period=1  dbl_ovrd=off  use_behavioral_HDL=off  implementation=Fabric  block_type=counter
  Slice : xbsIndex_r4/Slice  nbits=6  boolean_output=off  mode=Upper Bit Location + Width  bit1=0  base1=MSB of Input  bit0=0  base0=LSB of Input  dbl_ovrd=off  block_type=slice
  bram_din_const : xbsIndex_r4/Constant  const=0  gui_display_data_type=Fixed-point  arith_type=Signed (2's comp)  n_bits=18  bin_pt=17  preci_type=Single  exp_width=8  frac_width=24  explicit_period=off  period=1  equ=P=C  opselect=C  inp2=PCIN>>17  opr=+  inp1=P  carry=CIN  dbl_ovrd=off  block_type=constant
  bram_we_const : xbsIndex_r4/Constant  const=0  gui_display_data_type=Fixed-point  arith_type=Boolean  n_bits=16  bin_pt=14  preci_type=Single  exp_width=8  frac_width=24  explicit_period=off  period=1  equ=P=C  opselect=C  inp2=PCIN>>17  opr=+  inp1=P  carry=CIN  dbl_ovrd=off  block_type=constant
  cnt_sign_exta : xbsIndex_r4/Convert  gui_display_data_type=Fixed-point  arith_type=Unsigned  n_bits=10  bin_pt=0  float_type=Single  exp_bits=8  fraction_bits=24  quantization=Truncate  overflow=Wrap  en=off  latency=0  dbl_ovrd=off  pipeline=off  block_type=convert
  cnt_sign_extb : xbsIndex_r4/Convert  gui_display_data_type=Fixed-point  arith_type=Unsigned  n_bits=9  bin_pt=0  float_type=Single  exp_bits=8  fraction_bits=24  quantization=Truncate  overflow=Wrap  en=off  latency=0  dbl_ovrd=off  pipeline=off  block_type=convert
  coeff_mem : xbsIndex_r4/Dual Port RAM  depth=1024  initVector=[1 0.999076843261719 0.996315002441406 0.991706848144531 0.985275268554688 0.977027893066406 0.96697998046875 0.95513916015625 0.941543579101562 0.92620849609375 0.909164428710938 0.890449523925781 0.870086669921875 0.848121643066406 0.824592590332031 0.799537658691406 0.77301025390625 0.74505615234375 0.715728759765625 0.685081481933594 0.653175354003906 0.62005615234375 0.585800170898438 0.550460815429688 0.51409912109375 0.476799011230469 0.438613891601562 0.399627685546875 0.359893798828125 0.319503784179688 0.278518676757812 0.237022399902344 0.195091247558594 0.152793884277344 0.110221862792969 0.06744384765625 0.0245437622070312 -0.0184097290039062 -0.0613174438476562 -0.104118347167969 -0.146728515625 -0.189071655273438 -0.231056213378906 -0.272621154785156 -0.313682556152344 -0.354164123535156 -0.393989562988281 -0.433090209960938 -0.471397399902344 -0.508827209472656 -0.545326232910156 -0.580810546875 -0.615234375 -0.648513793945312 -0.68060302734375 -0.711433410644531 -0.740951538085938 -0.76910400390625 -0.79583740234375 -0.82110595703125 -0.844856262207031 -0.867042541503906 -0.887641906738281 -0.906593322753906 0 0 0 0 0 0 0 0 0 0 0 0 0 0 0 0 0 0 0 0 0 0 0 0 0 0 0 0 0 0 0 0 0 0 0 0 0 0 0 0 0 0 0 0 0 0 0 0 0 0 0 0 0 0 0 0 0 0 0 0 0 0 0 0 0 0 0 0 0 0 0 0 0 0 0 0 0 0 0 0 0 0 0 0 0 0 0 0 0 0 0 0 0 0 0 0 0 0 0 0 0 0 0 0 0 0 0 0 0 0 0 0 0 0 0 0 0 0 0 0 0 0 0 0 0 0 0 0 0 0 0 0 0 0 0 0 0 0 0 0 0 0 0 0 0 0 0 0 0 0 0 0 0 0 0 0 0 0 0 0 0 0 0 0 0 0 0 0 0 0 0 0 0 0 0 0 0 0 0 0 0 0 0 0 0 0 0 0 0 0 0 0 0 0 0 0 0 0 0 0 0 0 0 0 0 0 0 0 0 0 0 0 0 0 0 0 0 0 0 0 0 0 0 0 0 0 0 0 0 0 0 0 0 0 0 0 0 0 0 0 0 0 0 0 0 0 0 0 0 0 0 0 0 0 0 0 0 0 0 0 0 0 0 0 0 0 0 0 0 0 0 0 0 0 0 0 0 0 0 0 0 0 0 0 0 0 0 0 0 0 0 0 0 0 0 0 0 0 0 0 0 0 0 0 0 0 0 0 0 0 0 0 0 0 0 0 0 0 0 0 0 0 0 0 0 0 0 0 0 0 0 0 0 0 0 0 0 0 0 0 0 0 0 0 0 0 0 0 0 0 0 0 0 0 0 0 0 0 0 0 0 0 0 0 0 0 0 0 0 0 0 0 0 0 0 0 0 0 0 0 0 0 0 0 0 0 0 0 0 0 0 0 0 0 0 0 0 0 0 0 0 0 0 0 0 0 0 0 0 0 0 0 0 0 0 0 0 0 0 0 0 0 0 0 0 0 0 0 0 0 0 0 0 0 0 0 0 0 0 0 0 0 0 0 0 0 0 0 0 -0.042938232421875 -0.0858001708984375 -0.128501892089844 -0.17095947265625 -0.213111877441406 -0.254867553710938 -0.296150207519531 -0.336891174316406 -0.377006530761719 -0.416427612304688 -0.455085754394531 -0.492897033691406 -0.529800415039062 -0.56573486328125 -0.600616455078125 -0.634391784667969 -0.666999816894531 -0.698379516601562 -0.728462219238281 -0.757209777832031 -0.784553527832031 -0.810455322265625 -0.834861755371094 -0.85772705078125 -0.879013061523438 -0.898674011230469 -0.916679382324219 -0.932991027832031 -0.947586059570312 -0.960433959960938 -0.971504211425781 -0.980781555175781 -0.988258361816406 -0.993904113769531 -0.997726440429688 -0.999702453613281 -0.999832153320312 -0.998115539550781 -0.99456787109375 -0.989173889160156 -0.981964111328125 -0.972938537597656 -0.962120056152344 -0.949531555175781 -0.9351806640625 -0.919113159179688 -0.901351928710938 -0.881919860839844 -0.860870361328125 -0.838226318359375 -0.814033508300781 -0.788345336914062 -0.761199951171875 -0.732650756835938 -0.702751159667969 -0.671562194824219 -0.639122009277344 -0.605514526367188 -0.570777893066406 -0.534996032714844 -0.49822998046875 -0.460540771484375 -0.4219970703125 0 0 0 0 0 0 0 0 0 0 0 0 0 0 0 0 0 0 0 0 0 0 0 0 0 0 0 0 0 0 0 0 0 0 0 0 0 0 0 0 0 0 0 0 0 0 0 0 0 0 0 0 0 0 0 0 0 0 0 0 0 0 0 0 0 0 0 0 0 0 0 0 0 0 0 0 0 0 0 0 0 0 0 0 0 0 0 0 0 0 0 0 0 0 0 0 0 0 0 0 0 0 0 0 0 0 0 0 0 0 0 0 0 0 0 0 0 0 0 0 0 0 0 0 0 0 0 0 0 0 0 0 0 0 0 0 0 0 0 0 0 0 0 0 0 0 0 0 0 0 0 0 0 0 0 0 0 0 0 0 0 0 0 0 0 0 0 0 0 0 0 0 0 0 0 0 0 0 0 0 0 0 0 0 0 0 0 0 0 0 0 0 0 0 0 0 0 0 0 0 0 0 0 0 0 0 0 0 0 0 0 0 0 0 0 0 0 0 0 0 0 0 0 0 0 0 0 0 0 0 0 0 0 0 0 0 0 0 0 0 0 0 0 0 0 0 0 0 0 0 0 0 0 0 0 0 0 0 0 0 0 0 0 0 0 0 0 0 0 0 0 0 0 0 0 0 0 0 0 0 0 0 0 0 0 0 0 0 0 0 0 0 0 0 0 0 0 0 0 0 0 0 0 0 0 0 0 0 0 0 0 0 0 0 0 0 0 0 0 0 0 0 0 0 0 0 0 0 0 0 0 0 0 0 0 0 0 0 0 0 0 0 0 0 0 0 0 0 0 0 0 0 0 0 0 0 0 0 0 0 0 0 0 0 0 0 0 0 0 0 0 0 0 0 0 0 0 0 0 0 0 0 0 0 0 0 0 0 0 0 0 0 0 0 0 0 0 0 0 0 0 0 0 0 0 0 0 0 0 0 0 0 0 0 0 0 0 0 0 0 0 0 0 0 0 0 0 0 0 0 0 0 0 0 0 0 0 0 0 0 0 0 0 0 0 0 0 0]  distributed_mem=Block RAM  init_a=0  init_b=0  rst_a=off  rst_b=off  en_a=off  en_b=off  latency=2  write_mode_A=Read After Write  write_mode_B=Read After Write  dbl_ovrd=off  optimize=Area  use_rpm=on  block_type=dpram
  counter_b_concat : xbsIndex_r4/Concat  num_inputs=2  dbl_ovrd=off  block_type=concat
  counter_b_pad : xbsIndex_r4/Constant  const=1  gui_display_data_type=Fixed-point  arith_type=Unsigned  n_bits=1  bin_pt=0  preci_type=Single  exp_width=8  frac_width=24  explicit_period=off  period=1  equ=P=C  opselect=C  inp2=PCIN>>17  opr=+  inp1=P  carry=CIN  dbl_ovrd=off  block_type=constant
  ri_to_c : Subsystem
  w : Outport
  wires:
  Slice/1 -> cnt_sign_extb/1, cnt_sign_exta/1
  bram_din_const/1 -> coeff_mem/5, coeff_mem/2
  bram_we_const/1 -> coeff_mem/6, coeff_mem/3
  ri_to_c/1(c) -> w/1
  coeff_mem/2 -> ri_to_c/2(im)
  coeff_mem/1 -> ri_to_c/1(re)
  counter_b_concat/1 -> coeff_mem/4
  cnt_sign_exta/1 -> coeff_mem/1
  cnt_sign_extb/1 -> counter_b_concat/2
  counter_b_pad/1 -> counter_b_concat/1
  Counter/1 -> Slice/1
  rst/1 -> Counter/1

== system fft_wideband_real/fft_wideband_real/phase_mult/phase9_coeffs ==
  rst : Inport
  Counter : xbsIndex_r4/Counter  cnt_type=Free Running  cnt_to=Inf  operation=Up  start_count=0  cnt_by_val=1  arith_type=Unsigned  n_bits=6  bin_pt=0  load_pin=off  rst=on  en=off  explicit_period=on  period=1  dbl_ovrd=off  use_behavioral_HDL=off  implementation=Fabric  block_type=counter
  Slice : xbsIndex_r4/Slice  nbits=6  boolean_output=off  mode=Upper Bit Location + Width  bit1=0  base1=MSB of Input  bit0=0  base0=LSB of Input  dbl_ovrd=off  block_type=slice
  bram_din_const : xbsIndex_r4/Constant  const=0  gui_display_data_type=Fixed-point  arith_type=Signed (2's comp)  n_bits=18  bin_pt=17  preci_type=Single  exp_width=8  frac_width=24  explicit_period=off  period=1  equ=P=C  opselect=C  inp2=PCIN>>17  opr=+  inp1=P  carry=CIN  dbl_ovrd=off  block_type=constant
  bram_we_const : xbsIndex_r4/Constant  const=0  gui_display_data_type=Fixed-point  arith_type=Boolean  n_bits=16  bin_pt=14  preci_type=Single  exp_width=8  frac_width=24  explicit_period=off  period=1  equ=P=C  opselect=C  inp2=PCIN>>17  opr=+  inp1=P  carry=CIN  dbl_ovrd=off  block_type=constant
  cnt_sign_exta : xbsIndex_r4/Convert  gui_display_data_type=Fixed-point  arith_type=Unsigned  n_bits=10  bin_pt=0  float_type=Single  exp_bits=8  fraction_bits=24  quantization=Truncate  overflow=Wrap  en=off  latency=0  dbl_ovrd=off  pipeline=off  block_type=convert
  cnt_sign_extb : xbsIndex_r4/Convert  gui_display_data_type=Fixed-point  arith_type=Unsigned  n_bits=9  bin_pt=0  float_type=Single  exp_bits=8  fraction_bits=24  quantization=Truncate  overflow=Wrap  en=off  latency=0  dbl_ovrd=off  pipeline=off  block_type=convert
  coeff_mem : xbsIndex_r4/Dual Port RAM  depth=1024  initVector=[1 0.998794555664062 0.995185852050781 0.989173889160156 0.980781555175781 0.97003173828125 0.956939697265625 0.941543579101562 0.923881530761719 0.90399169921875 0.881919860839844 0.85772705078125 0.831466674804688 0.803207397460938 0.77301025390625 0.740951538085938 0.707107543945312 0.671562194824219 0.634391784667969 0.595695495605469 0.555572509765625 0.51409912109375 0.471397399902344 0.427558898925781 0.382682800292969 0.336891174316406 0.290283203125 0.24298095703125 0.195091247558594 0.146728515625 0.0980148315429688 0.0490646362304688 0 -0.0490646362304688 -0.0980148315429688 -0.146728515625 -0.195091247558594 -0.24298095703125 -0.290283203125 -0.336891174316406 -0.382682800292969 -0.427558898925781 -0.471397399902344 -0.51409912109375 -0.555572509765625 -0.595695495605469 -0.634391784667969 -0.671562194824219 -0.707107543945312 -0.740951538085938 -0.77301025390625 -0.803207397460938 -0.831466674804688 -0.85772705078125 -0.881919860839844 -0.90399169921875 -0.923881530761719 -0.941543579101562 -0.956939697265625 -0.97003173828125 -0.980781555175781 -0.989173889160156 -0.995185852050781 -0.998794555664062 0 0 0 0 0 0 0 0 0 0 0 0 0 0 0 0 0 0 0 0 0 0 0 0 0 0 0 0 0 0 0 0 0 0 0 0 0 0 0 0 0 0 0 0 0 0 0 0 0 0 0 0 0 0 0 0 0 0 0 0 0 0 0 0 0 0 0 0 0 0 0 0 0 0 0 0 0 0 0 0 0 0 0 0 0 0 0 0 0 0 0 0 0 0 0 0 0 0 0 0 0 0 0 0 0 0 0 0 0 0 0 0 0 0 0 0 0 0 0 0 0 0 0 0 0 0 0 0 0 0 0 0 0 0 0 0 0 0 0 0 0 0 0 0 0 0 0 0 0 0 0 0 0 0 0 0 0 0 0 0 0 0 0 0 0 0 0 0 0 0 0 0 0 0 0 0 0 0 0 0 0 0 0 0 0 0 0 0 0 0 0 0 0 0 0 0 0 0 0 0 0 0 0 0 0 0 0 0 0 0 0 0 0 0 0 0 0 0 0 0 0 0 0 0 0 0 0 0 0 0 0 0 0 0 0 0 0 0 0 0 0 0 0 0 0 0 0 0 0 0 0 0 0 0 0 0 0 0 0 0 0 0 0 0 0 0 0 0 0 0 0 0 0 0 0 0 0 0 0 0 0 0 0 0 0 0 0 0 0 0 0 0 0 0 0 0 0 0 0 0 0 0 0 0 0 0 0 0 0 0 0 0 0 0 0 0 0 0 0 0 0 0 0 0 0 0 0 0 0 0 0 0 0 0 0 0 0 0 0 0 0 0 0 0 0 0 0 0 0 0 0 0 0 0 0 0 0 0 0 0 0 0 0 0 0 0 0 0 0 0 0 0 0 0 0 0 0 0 0 0 0 0 0 0 0 0 0 0 0 0 0 0 0 0 0 0 0 0 0 0 0 0 0 0 0 0 0 0 0 0 0 0 0 0 0 0 0 0 0 0 0 0 0 0 0 0 0 0 0 0 0 0 0 0 0 0 0 0 0 0 0 0 0 0 0 0 0 0 0 -0.0490646362304688 -0.0980148315429688 -0.146728515625 -0.195091247558594 -0.24298095703125 -0.290283203125 -0.336891174316406 -0.382682800292969 -0.427558898925781 -0.471397399902344 -0.51409912109375 -0.555572509765625 -0.595695495605469 -0.634391784667969 -0.671562194824219 -0.707107543945312 -0.740951538085938 -0.77301025390625 -0.803207397460938 -0.831466674804688 -0.85772705078125 -0.881919860839844 -0.90399169921875 -0.923881530761719 -0.941543579101562 -0.956939697265625 -0.97003173828125 -0.980781555175781 -0.989173889160156 -0.995185852050781 -0.998794555664062 -1 -0.998794555664062 -0.995185852050781 -0.989173889160156 -0.980781555175781 -0.97003173828125 -0.956939697265625 -0.941543579101562 -0.923881530761719 -0.90399169921875 -0.881919860839844 -0.85772705078125 -0.831466674804688 -0.803207397460938 -0.77301025390625 -0.740951538085938 -0.707107543945312 -0.671562194824219 -0.634391784667969 -0.595695495605469 -0.555572509765625 -0.51409912109375 -0.471397399902344 -0.427558898925781 -0.382682800292969 -0.336891174316406 -0.290283203125 -0.24298095703125 -0.195091247558594 -0.146728515625 -0.0980148315429688 -0.0490646362304688 0 0 0 0 0 0 0 0 0 0 0 0 0 0 0 0 0 0 0 0 0 0 0 0 0 0 0 0 0 0 0 0 0 0 0 0 0 0 0 0 0 0 0 0 0 0 0 0 0 0 0 0 0 0 0 0 0 0 0 0 0 0 0 0 0 0 0 0 0 0 0 0 0 0 0 0 0 0 0 0 0 0 0 0 0 0 0 0 0 0 0 0 0 0 0 0 0 0 0 0 0 0 0 0 0 0 0 0 0 0 0 0 0 0 0 0 0 0 0 0 0 0 0 0 0 0 0 0 0 0 0 0 0 0 0 0 0 0 0 0 0 0 0 0 0 0 0 0 0 0 0 0 0 0 0 0 0 0 0 0 0 0 0 0 0 0 0 0 0 0 0 0 0 0 0 0 0 0 0 0 0 0 0 0 0 0 0 0 0 0 0 0 0 0 0 0 0 0 0 0 0 0 0 0 0 0 0 0 0 0 0 0 0 0 0 0 0 0 0 0 0 0 0 0 0 0 0 0 0 0 0 0 0 0 0 0 0 0 0 0 0 0 0 0 0 0 0 0 0 0 0 0 0 0 0 0 0 0 0 0 0 0 0 0 0 0 0 0 0 0 0 0 0 0 0 0 0 0 0 0 0 0 0 0 0 0 0 0 0 0 0 0 0 0 0 0 0 0 0 0 0 0 0 0 0 0 0 0 0 0 0 0 0 0 0 0 0 0 0 0 0 0 0 0 0 0 0 0 0 0 0 0 0 0 0 0 0 0 0 0 0 0 0 0 0 0 0 0 0 0 0 0 0 0 0 0 0 0 0 0 0 0 0 0 0 0 0 0 0 0 0 0 0 0 0 0 0 0 0 0 0 0 0 0 0 0 0 0 0 0 0 0 0 0 0 0 0 0 0 0 0 0 0 0 0 0 0 0 0 0 0 0 0 0 0 0 0 0 0 0 0 0 0 0 0 0 0 0 0 0 0 0 0 0 0 0 0 0 0 0 0 0 0 0 0 0 0 0]  distributed_mem=Block RAM  init_a=0  init_b=0  rst_a=off  rst_b=off  en_a=off  en_b=off  latency=2  write_mode_A=Read After Write  write_mode_B=Read After Write  dbl_ovrd=off  optimize=Area  use_rpm=on  block_type=dpram
  counter_b_concat : xbsIndex_r4/Concat  num_inputs=2  dbl_ovrd=off  block_type=concat
  counter_b_pad : xbsIndex_r4/Constant  const=1  gui_display_data_type=Fixed-point  arith_type=Unsigned  n_bits=1  bin_pt=0  preci_type=Single  exp_width=8  frac_width=24  explicit_period=off  period=1  equ=P=C  opselect=C  inp2=PCIN>>17  opr=+  inp1=P  carry=CIN  dbl_ovrd=off  block_type=constant
  ri_to_c : Subsystem
  w : Outport
  wires:
  Slice/1 -> cnt_sign_extb/1, cnt_sign_exta/1
  bram_din_const/1 -> coeff_mem/5, coeff_mem/2
  bram_we_const/1 -> coeff_mem/6, coeff_mem/3
  ri_to_c/1(c) -> w/1
  coeff_mem/2 -> ri_to_c/2(im)
  coeff_mem/1 -> ri_to_c/1(re)
  counter_b_concat/1 -> coeff_mem/4
  cnt_sign_exta/1 -> coeff_mem/1
  cnt_sign_extb/1 -> counter_b_concat/2
  counter_b_pad/1 -> counter_b_concat/1
  Counter/1 -> Slice/1
  rst/1 -> Counter/1

== system fft_wideband_real/fft_wideband_real/to_workspace_complex16/c_to_ri ==
  c : Inport
  force_im : xbsIndex_r4/Reinterpret  force_arith_type=on  arith_type="Signed  (2's comp)"  force_bin_pt=on  bin_pt=17  block_type=reinterpret
  force_re : xbsIndex_r4/Reinterpret  force_arith_type=on  arith_type="Signed  (2's comp)"  force_bin_pt=on  bin_pt=17  block_type=reinterpret
  slice_im : xbsIndex_r4/Slice  nbits=18  boolean_output=off  mode=Lower Bit Location + Width  bit1=0  base1=MSB of Input  bit0=0  base0=LSB of Input  dbl_ovrd=off  block_type=slice
  slice_re : xbsIndex_r4/Slice  nbits=18  boolean_output=off  mode=Upper Bit Location + Width  bit1=0  base1=MSB of Input  bit0=0  base0=LSB of Input  dbl_ovrd=off  block_type=slice
  re : Outport
  im : Outport  Port=2
  wires:
  c/1 -> slice_im/1, slice_re/1
  force_im/1 -> im/1
  slice_im/1 -> force_im/1
  force_re/1 -> re/1
  slice_re/1 -> force_re/1
